simulink model "ScaraRobotApresentacao2023"  (R2024a)
settings: Solver=VariableStepAuto  StartTime=0.0  StopTime=200  RelTol=1e-3
model workspace: external: MATLAB File C:\Users\lucas\OneDrive\Documents\MATLAB\Robotica_2023b\ScaraRobot_DataFile.m (data not in the file)
values from neighbouring files (symbols this model uses):
  I = cell(1,n)    [calcularDinamica.m]    (also in inicializacaoAntropomorfico.m = {I1, I2, I3, I4, I5, I6, I7})
  L = [L1, L2, L3, L4, L5, L6, L7]    [inicializacaoAntropomorfico.m]
  Lcm = {Lcm1, Lcm2, Lcm3, Lcm4, Lcm5, Lcm6, Lcm7}    [inicializacaoAntropomorfico.m]
  m = [m1, m2, m3, m4, m5, m6, m7]    [inicializacaoAntropomorfico.m]
  Pf = [  0.05    [inicializacaoAntropomorfico.m]
  Pi = [  0.2    [inicializacaoAntropomorfico.m]
  Raio = [0]    [inicializacaoAntropomorfico.m]
  Sentido = [0]    [inicializacaoAntropomorfico.m]
  Tipo = [1]    [inicializacaoAntropomorfico.m]
undefined symbols (not defined in the file or in its folder): Lx1, Lx2, smiData, X, Y, Z
libraries: sm_lib x25, nesl_utility x5
(part 10 of 10)

== matlab function ScaraRobotApresentacao2023/Control ==
  data: M input; Tc output; H input; G input; C input; Qd input; dQd input; d2Qd input; Q input; dQ input
function Tc = Controlador(M, H, G, C, Qd, dQd, d2Qd, Q, dQ)

    g  = 9.81;
    KP = kp * eye(6);            % Ganho proporcional
    KD = 2 * sqrt(kp) * eye(6);  % Ganho derivativo
    erro = Qd - Q;
    erro_dot = dQd - dQ;
    Tc = M * (d2Qd + KD * erro_dot + KP * erro) + H + C + G;

== matlab function ScaraRobotApresentacao2023/Plant ==
  data: M input; H input; G input; C input; Tc input; d2Q output
function d2Q  = planta(M,H,G,C,Tc)
    d2Q = zeros(4,1);
    d2Q = M\(Tc-H-C-G);
end
